simulink model "CollisionAvoidance_Demo"  (R2019a)
settings: Solver=VariableStepAuto  StartTime=0.0  StopTime=200  RelTol=1e-3
values from neighbouring files (symbols this model uses):
  p1x_goal = 100    [simin.m]    (also in simin.mat)
  p1x_ini = 100    [simin.m]    (also in simin.mat)
  p1y_goal = 200    [simin.m]    (also in simin.mat)
  p1y_ini = 0    [simin.m]    (also in simin.mat)
  p2x_ini = 0    [simin.m]    (also in simin.mat)
  p2y_ini = 100    [simin.m]    (also in simin.mat)
  r1 = 10    [simin.m]    (also in simin.mat)
  r2 = 10    [simin.m]    (also in simin.mat)
  v1x_ini = v_ref * (p1x_goal - p1x_ini) / (sqrt( (p1x_goal - p1x_ini)^2 + (p1y_goal - p1y_ini)^2) )    [simin.m]    (also in simin.mat = 0)
  v1y_ini = v_ref * (p1y_goal - p1y_ini) / (sqrt( (p1x_goal - p1x_ini)^2 + (p1y_goal - p1y_ini)^2) )    [simin.m]    (also in simin.mat = 1)
  v2x_ini = 1.0    (= 1)    [simin.m]    (also in simin.mat)
  v2y_ini = 0.0    (= 0)    [simin.m]    (also in simin.mat)
  v_ref = 1.0    (= 1)    [simin.m]    (also in simin.mat)
undefined symbols (not defined in the file or in its folder): v_init
settings Model: Creator=kocab  LastModifiedBy=kocab

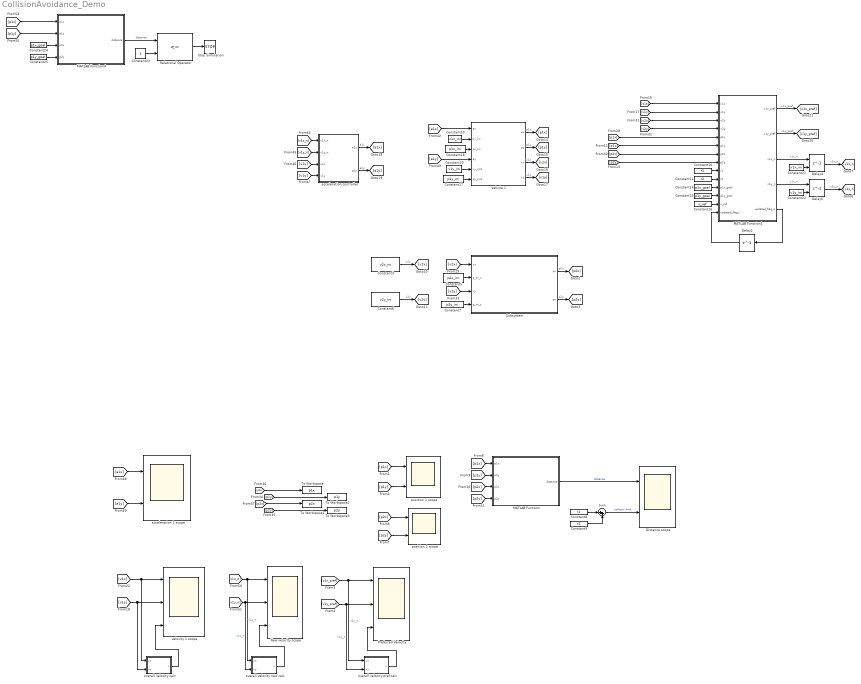
== system CollisionAvoidance_Demo ==
  Constant10 : Constant  Value=r1
  Constant11 : Constant  Value=r2
  Constant14 : Constant  Value=p1x_goal
  Constant15 : Constant  Value=p1y_goal
  Constant16 : Constant  Value=v_ref
  Constant17 : Constant  Value=p1y_ini
  Constant18 : Constant  Value=p1x_ini
  Constant19 : Constant  Value=v1x_ini
  Constant20 : Constant  Value=v1y_ini
  Constant21 : Constant  Value=v1x_ini
  Constant22 : Constant  Value=v1y_ini
  Constant23 : Constant
  Constant24 : Constant  Value=p1x_goal
  Constant25 : Constant  Value=p1y_goal
  Constant3 : Constant  Value=v2x_ini
  Constant5 : Constant  Value=p2x_ini
  Constant6 : Constant  Value=v2y_ini
  Constant7 : Constant  Value=p2y_ini
  Constant8 : Constant  Value=r1
  Constant9 : Constant  Value=r2
  Delay2 : Delay  DelayLength=1  InitialCondition=0
  Delay4 : Delay  DelayLength=1  InitialConditionSource=Input port
      settings: InputPortMap=u0,p4
  Delay5 : Delay  DelayLength=1  InitialConditionSource=Input port
      settings: InputPortMap=u0,p4
  Distance scope : Scope  NumInputPorts=2
  MATLAB Function : MATLAB Function  TreatAsAtomicUnit=on
  MATLAB Function1 : MATLAB Function  TreatAsAtomicUnit=on
  MATLAB Function4 : MATLAB Function  TreatAsAtomicUnit=on
  New velocity scope : Scope  NumInputPorts=3
  Preferred Velocity : Scope  NumInputPorts=3
  Relational Operator : RelationalOperator  Operator=<=  OutDataTypeStr=boolean  RndMeth=Simplest
  Stop Simulation : Stop
  Subsystem : Subsystem
  Sum : Sum  Inputs=|++
  To Workspace : ToWorkspace  VariableName=p1x  SampleTime=-1
  To Workspace1 : ToWorkspace  VariableName=p2x  SampleTime=-1
  To Workspace2 : ToWorkspace  VariableName=p1y  SampleTime=-1
  To Workspace3 : ToWorkspace  VariableName=p2y  SampleTime=-1
  Vehicle 1 : Subsystem
  acceleration 1 scope : Scope  NumInputPorts=2
  acceleration controller : MATLAB Function  TreatAsAtomicUnit=on
  overall velocity calc : MATLAB Function  TreatAsAtomicUnit=on
  overall velocity new calc : MATLAB Function  TreatAsAtomicUnit=on
  overall velocity pref calc : MATLAB Function  TreatAsAtomicUnit=on
  "position 1 scope " : Scope  NumInputPorts=2
  position 2 scope : Scope  NumInputPorts=2
  velocity 1 scope : Scope  NumInputPorts=3
  wires:
  Subsystem/1(px) -> [p2x]  "p2x"
  Constant3/1 -> [v2x]  "v2x"
  Constant5/1 -> Subsystem/2(p_ini_x)
  Constant6/1 -> [v2y]  "v2y"
  Constant7/1 -> Subsystem/4(p_ini_y)
  Subsystem/2(py) -> [p2y]  "p2y"
  [p1x] -> "position 1 scope "/1
  [p1y] -> "position 1 scope "/2
  [p2y] -> position 2 scope/2
  [p2x] -> position 2 scope/1
  [p1x] -> MATLAB Function/1(p1x)
  [p1y] -> MATLAB Function/2(p1y)
  [p2x] -> MATLAB Function/3(p2x)
  [p2y] -> MATLAB Function/4(p2y)
  MATLAB Function/1(distance) -> Distance scope/1  "distance"
  Constant9/1 -> Sum/2
  Constant8/1 -> Sum/1
  Sum/1 -> Distance scope/2  "collision limit"
  Constant10/1 -> MATLAB Function1/9(r1)
  [p1y] -> MATLAB Function1/6(p1y)
  [v1y] -> MATLAB Function1/2(v1y)
  [v1x] -> MATLAB Function1/1(v1x)
  [p2y] -> MATLAB Function1/8(p2y)
  Constant11/1 -> MATLAB Function1/10(r2)
  MATLAB Function1/3(v1x_n) -> Delay4/1  "v1x_n"
  Delay5/1 -> [v1y_n]  "v1y_n"
  [v1y] -> velocity 1 scope/2, overall velocity calc/2(vy)
  [v1x] -> overall velocity calc/1(vx), velocity 1 scope/1
  Delay2/1 -> MATLAB Function1/14(updated_flag_i)
  MATLAB Function1/5(updated_flag_o) -> Delay2/1
  [p1x] -> MATLAB Function1/5(p1x)
  [p2x] -> MATLAB Function1/7(p2x)
  [v2x] -> MATLAB Function1/3(v2x)
  [v2y] -> MATLAB Function1/4(v2y)
  [v2x] -> Subsystem/1(vx)
  [v2y] -> Subsystem/3(vy)
  [p1x] -> To Workspace/1
  [p2x] -> To Workspace1/1
  [p1y] -> To Workspace2/1
  [p2y] -> To Workspace3/1
  Constant14/1 -> MATLAB Function1/11(p1x_goal)
  Constant15/1 -> MATLAB Function1/12(p1y_goal)
  Constant16/1 -> MATLAB Function1/13(v_ref)
  [a1y] -> Vehicle 1/4(ay)
  [a1x] -> Vehicle 1/1(ax)
  Constant17/1 -> Vehicle 1/6(py_ini1)
  Constant18/1 -> Vehicle 1/3(px_ini)
  Constant20/1 -> Vehicle 1/5(vy_ini1)
  Constant19/1 -> Vehicle 1/2(vx_ini)
  Vehicle 1/1(px) -> [p1x]  "p1x"
  Vehicle 1/2(py) -> [p1y]  "p1y"
  Vehicle 1/3(vx) -> [v1x]  "v1x"
  Vehicle 1/4(vy) -> [v1y]  "v1y"
  acceleration controller/1(a1x) -> [a1x]  "a1x"
  [v1x_n] -> acceleration controller/1(v1x_n)
  [v1y_n] -> acceleration controller/2(v1y_n)
  [v1x] -> acceleration controller/3(v1x)
  [v1y] -> acceleration controller/4(v1y)
  [a1x] -> acceleration 1 scope/1
  [a1y] -> acceleration 1 scope/2
  [v1y_n] -> overall velocity new calc/2(vy), New velocity scope/2  "v1y_n"
  [v1x_n] -> overall velocity new calc/1(vx), New velocity scope/1  "v1x_n"
  acceleration controller/2(a1y) -> [a1y]  "a1y"
  Constant21/1 -> Delay4/2
  Delay4/1 -> [v1x_n]  "v1x_n"
  MATLAB Function1/4(v1y_n) -> Delay5/1  "v1x_n"
  Constant22/1 -> Delay5/2
  MATLAB Function4/1(distance) -> Relational Operator/1  "distance"
  Constant23/1 -> Relational Operator/2
  [p1x] -> MATLAB Function4/1(p1x)
  [p1y] -> MATLAB Function4/2(p1y)
  Constant24/1 -> MATLAB Function4/3(p2x)
  Constant25/1 -> MATLAB Function4/4(p2y)
  Relational Operator/1 -> Stop Simulation/1
  overall velocity calc/1(v) -> velocity 1 scope/3
  MATLAB Function1/1(v1x_pref) -> [v1x_pref]  "v1x_pref"
  MATLAB Function1/2(v1y_pref) -> [v1y_pref]  "v1y_pref"
  overall velocity new calc/1(v) -> New velocity scope/3
  [v1x_pref] -> Preferred Velocity/1, overall velocity pref calc/1(vx)  "v1x_n"
  overall velocity pref calc/1(v) -> Preferred Velocity/3
  [v1y_pref] -> overall velocity pref calc/2(vy), Preferred Velocity/2  "v1y_n"

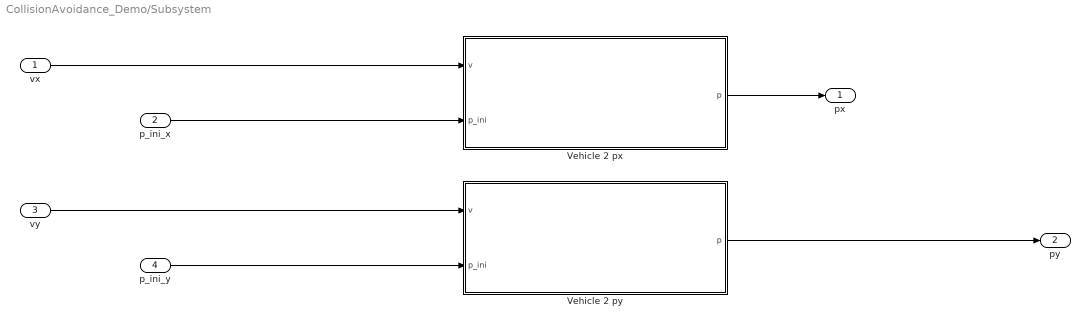
== system CollisionAvoidance_Demo/Subsystem ==
  vx : Inport
  p_ini_x : Inport  Port=2
  vy : Inport  Port=3
  p_ini_y : Inport  Port=4
  Vehicle 2 px : Subsystem
  Vehicle 2 py : Subsystem
  px : Outport
  py : Outport  Port=2
  wires:
  p_ini_y/1 -> Vehicle 2 py/2(p_ini)
  vx/1 -> Vehicle 2 px/1(v)
  vy/1 -> Vehicle 2 py/1(v)
  p_ini_x/1 -> Vehicle 2 px/2(p_ini)
  Vehicle 2 px/1(p) -> px/1
  Vehicle 2 py/1(p) -> py/1

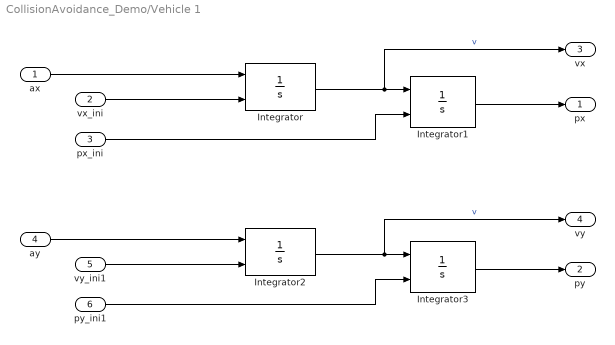
== system CollisionAvoidance_Demo/Vehicle 1 ==
  ax : Inport
  vx_ini : Inport  Port=2
  px_ini : Inport  Port=3
  ay : Inport  Port=4
  vy_ini1 : Inport  Port=5
  py_ini1 : Inport  Port=6
  Integrator : Integrator  InitialConditionSource=external  InitialCondition=v_init
  Integrator1 : Integrator  InitialConditionSource=external
  Integrator2 : Integrator  InitialConditionSource=external  InitialCondition=v_init
  Integrator3 : Integrator  InitialConditionSource=external
  px : Outport
  py : Outport  Port=2
  vx : Outport  Port=3
  vy : Outport  Port=4
  wires:
  ax/1 -> Integrator/1
  Integrator/1 -> vx/1, Integrator1/1  "v"
  px_ini/1 -> Integrator1/2
  vx_ini/1 -> Integrator/2
  Integrator1/1 -> px/1
  vy_ini1/1 -> Integrator2/2
  Integrator2/1 -> vy/1, Integrator3/1  "v"
  py_ini1/1 -> Integrator3/2
  ay/1 -> Integrator2/1
  Integrator3/1 -> py/1

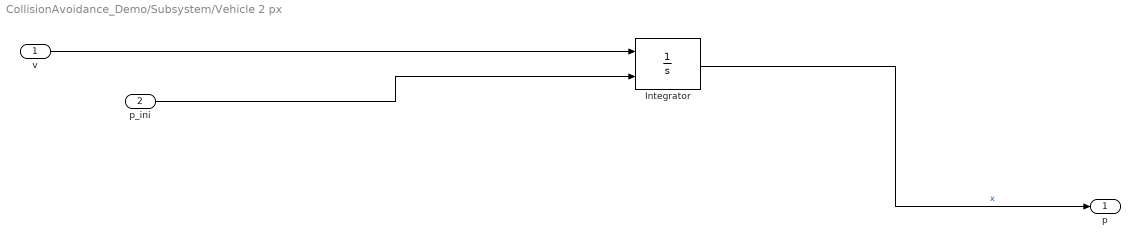
== system CollisionAvoidance_Demo/Subsystem/Vehicle 2 px ==
  v : Inport
  p_ini : Inport  Port=2
  Integrator : Integrator  InitialConditionSource=external
  p : Outport
  wires:
  p_ini/1 -> Integrator/2
  Integrator/1 -> p/1  "x"
  v/1 -> Integrator/1

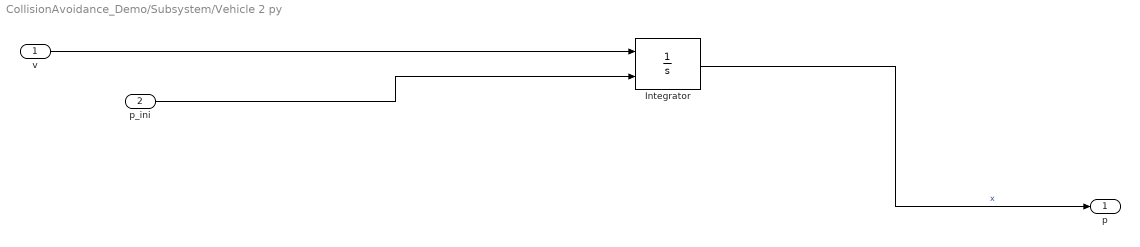
== system CollisionAvoidance_Demo/Subsystem/Vehicle 2 py ==
  v : Inport
  p_ini : Inport  Port=2
  Integrator : Integrator  InitialConditionSource=external
  p : Outport
  wires:
  p_ini/1 -> Integrator/2
  Integrator/1 -> p/1  "x"
  v/1 -> Integrator/1

== matlab function CollisionAvoidance_Demo/MATLAB Function1 ==
  data: v1x_pref output; v1y_pref output; v1x input; v1x_n output; v1y input; v2x input; v2y input; p1x input; p1y input; p2x input; p2y input; r1 input; r2 input; p1x_goal input; p1y_goal input; v_ref input; v1y_n output; updated_flag_i input; updated_flag_o output
function [v1x_pref, v1y_pref, v1x_n, v1y_n, updated_flag_o] = fcn(v1x, v1y, v2x, v2y, p1x, p1y, p2x, p2y, r1, r2, p1x_goal, p1y_goal, v_ref, updated_flag_i)
% compute preferred velocity
v1x_pref = v_ref * (p1x_goal - p1x) / (sqrt( (p1x_goal - p1x)^2 + (p1y_goal - p1y)^2) ) ;
v1y_pref = v_ref * (p1y_goal - p1y) / (sqrt( (p1x_goal - p1x)^2 + (p1y_goal - p1y)^2) ) ;
% margin
Theta_marg = 1.0 ;
%% Initialization
v1x_n = v1x_pref ;
v1y_n = v1y_pref ;
updated_flag_o = 0 ;


if (updated_flag_i == 1)
%     v1x_n = v1x_pref ;
%     v1y_n = v1y_pref ;
else
    %% Computation tangent to collision circle (for position graph)
    % Theta1 : angle( x-axis , line(p1,p2) )
    % Theta2 : angle( line(p1,p2) , tangents of collision circle)
    Theta1 = atan( (p2y - p1y) / (p2x - p1x) ) ;
    Theta2 = asin( (r1 + r2) / distance(p1x,p1y,p2x,p2y) ) * Theta_marg ;

    % m1 : slope of first tangent
    % m2 : slope of second tangent
    m1 = tan( Theta1 - Theta2 ) ;
    m2 = tan( Theta1 + Theta2 ) ;
    
    %% Computation new velocity (for velocity graph)
    % compute relative velocity
    v1x_rel = v1x_pref - v2x ;
    v1y_rel = v1y_pref - v2y ;
    % is relative velocity within collision limits
    isCollision = ((v1y_rel/v1x_rel) > m1) && ((v1y_rel/v1x_rel) < m2) ;
    % new velocity initialization
    v1x_n1 = 0 ;
    v1y_n1 = 0 ;
    v1x_n2 = 0 ;
    v1y_n2 = 0 ;
    if isCollision
        % option 1
        v1x_n1 = v2x + ( v1x_rel + (v1y_rel - m1 * v1x_rel) * m1 / (m1^2 + 1) ) ;
        v1y_n1 = v2y + ( v1y_rel - (v1y_rel - m1 * v1x_rel) / (m1^2 + 1) ) ;
        % option 2
        v1x_n2 = v2x + ( v1x_rel + (v1y_rel - m2 * v1x_rel) * m2 / (m2^2 + 1) ) ;
        v1y_n2 = v2y + ( v1y_rel - (v1y_rel - m2 * v1x_rel) / (m2^2 + 1) ) ;
            % choose nearest option
        if (distance(v1x_pref,v1y_pref,v1x_n1,v1y_n1) < distance(v1x_pref,v1y_pref,v1x_n2,v1y_n2))
            v1x_n = v1x_n1 ;
            v1y_n = v1y_n1 ;
        else
            v1x_n = v1x_n2 ;
            v1y_n = v1y_n2 ;
        end

    else
        % no velocity update
    end
end
end

== matlab function CollisionAvoidance_Demo/MATLAB Function ==
  data: p1x input; distance output; p1y input; p2x input; p2y input
function distance = distance(p1x,p1y,p2x,p2y)
    
distance = sqrt((p1x-p2x)^2+(p1y-p2y)^2);

== matlab function CollisionAvoidance_Demo/acceleration controller ==
  data: v1x_n input; a1x output; v1y_n input; a1y output; v1x input; v1y input
function [a1x, a1y] = fcn(v1x_n, v1y_n, v1x, v1y)
a1x = v1x_n - v1x ;
a1y = v1y_n - v1y ;

== matlab function CollisionAvoidance_Demo/MATLAB Function4 ==
  data: p1x input; distance output; p1y input; p2x input; p2y input
function distance = distance(p1x,p1y,p2x,p2y)
    
distance = sqrt((p1x-p2x)^2+(p1y-p2y)^2);

== matlab function CollisionAvoidance_Demo/overall velocity calc ==
  data: vx input; v output; vy input
function v = fcn(vx,vy)

v = sqrt( vx^2 + vy^2 ) ;

== matlab function CollisionAvoidance_Demo/overall velocity new calc ==
  data: vx input; v output; vy input
function v = fcn(vx,vy)

v = sqrt( vx^2 + vy^2 ) ;

== matlab function CollisionAvoidance_Demo/overall velocity pref calc ==
  data: vx input; v output; vy input
function v = fcn(vx,vy)

v = sqrt( vx^2 + vy^2 ) ;
